simulink model "c00014M_harness"  (R2018a)
settings: Solver=FixedStepAuto  StartTime=0.0  StopTime=300  FixedStep=0.1  RelTol=1e-3
undefined symbols (not defined in the file): A1, hmax, PriorityTank, R1, R2, sigbuilder_block
(part 5 of 24)

== system c00014M_harness/M184 ==
  note: VALUES
      | ---------------------------------
      | ControlType = 1 | 2 | 3
      | FillTank = 0 | 1
      | EmptyTank = 0 | 1
      | ManualReference between 0 and 1
      | Tempreature between 0 and 100
      | EmergencyButton = 0 | 1
      | LiquidLevel between 0 and 1 (hmax)
  note: Inputs For Tank2
  note: NAMES
      | --------------------------------------------
      | CT1 = ControlType Tank 1
      | F1 = Fill Tank 1
      | E1 = Empty Tank 1
      | MR1 = Manual Reference Tank1
      | T1 = Temperature Tank 1
      | EB1 = Emergency Button Tank 1
      | LL1 = Liquid Level 1
  note: Inputs For Tank3
  note: Inputs For Tank1
  CT1 : Inport
  F1 : Inport  Port=2
  E1 : Inport  Port=3
  T1 : Inport  Port=4
  EB1 : Inport  Port=5
  CT3 : Inport  Port=6
  T3 : Inport  Port=7
  EB3 : Inport  Port=8
  Tank1 : Subsystem
  Tank3 : Subsystem
  LL1 : Outport
  LL3 : Outport  Port=2
  wires:
  EB1/1 -> Tank1/5(EB1)
  Tank3/1(LL3) -> LL3/1, Tank1/6(LL3)
  T1/1 -> Tank1/4(T1)
  Tank1/1(LL1) -> LL1/1, Tank3/4(LL1)
  F1/1 -> Tank1/2(F1)
  E1/1 -> Tank1/3(E1)
  CT3/1 -> Tank3/1(CT3)
  EB3/1 -> Tank3/3(EB3)
  T3/1 -> Tank3/2(T3)
  CT1/1 -> Tank1/1(CT1)

== system c00014M_harness/M185 ==
  note: VALUES
      | ---------------------------------
      | ControlType = 1 | 2 | 3
      | FillTank = 0 | 1
      | EmptyTank = 0 | 1
      | ManualReference between 0 and 1
      | Tempreature between 0 and 100
      | EmergencyButton = 0 | 1
      | LiquidLevel between 0 and 1 (hmax)
  note: Inputs For Tank2
  note: NAMES
      | --------------------------------------------
      | CT1 = ControlType Tank 1
      | F1 = Fill Tank 1
      | E1 = Empty Tank 1
      | MR1 = Manual Reference Tank1
      | T1 = Temperature Tank 1
      | EB1 = Emergency Button Tank 1
      | LL1 = Liquid Level 1
  note: Inputs For Tank3
  note: Inputs For Tank1
  CT1 : Inport
  F1 : Inport  Port=2
  E1 : Inport  Port=3
  T1 : Inport  Port=4
  EB1 : Inport  Port=5
  CT3 : Inport  Port=6
  T3 : Inport  Port=7
  EB3 : Inport  Port=8
  Tank1 : Subsystem
  Tank3 : Subsystem
  LL1 : Outport
  LL3 : Outport  Port=2
  wires:
  EB1/1 -> Tank1/5(EB1)
  Tank3/1(LL3) -> LL3/1, Tank1/6(LL3)
  T1/1 -> Tank1/4(T1)
  Tank1/1(LL1) -> LL1/1, Tank3/4(LL1)
  F1/1 -> Tank1/2(F1)
  E1/1 -> Tank1/3(E1)
  CT3/1 -> Tank3/1(CT3)
  EB3/1 -> Tank3/3(EB3)
  T3/1 -> Tank3/2(T3)
  CT1/1 -> Tank1/1(CT1)

== system c00014M_harness/M186 ==
  note: VALUES
      | ---------------------------------
      | ControlType = 1 | 2 | 3
      | FillTank = 0 | 1
      | EmptyTank = 0 | 1
      | ManualReference between 0 and 1
      | Tempreature between 0 and 100
      | EmergencyButton = 0 | 1
      | LiquidLevel between 0 and 1 (hmax)
  note: Inputs For Tank2
  note: NAMES
      | --------------------------------------------
      | CT1 = ControlType Tank 1
      | F1 = Fill Tank 1
      | E1 = Empty Tank 1
      | MR1 = Manual Reference Tank1
      | T1 = Temperature Tank 1
      | EB1 = Emergency Button Tank 1
      | LL1 = Liquid Level 1
  note: Inputs For Tank3
  note: Inputs For Tank1
  CT1 : Inport
  F1 : Inport  Port=2
  E1 : Inport  Port=3
  T1 : Inport  Port=4
  EB1 : Inport  Port=5
  CT3 : Inport  Port=6
  T3 : Inport  Port=7
  EB3 : Inport  Port=8
  Tank1 : Subsystem
  Tank3 : Subsystem
  LL1 : Outport
  LL3 : Outport  Port=2
  wires:
  EB1/1 -> Tank1/5(EB1)
  Tank3/1(LL3) -> LL3/1, Tank1/6(LL3)
  T1/1 -> Tank1/4(T1)
  Tank1/1(LL1) -> LL1/1, Tank3/4(LL1)
  F1/1 -> Tank1/2(F1)
  E1/1 -> Tank1/3(E1)
  CT3/1 -> Tank3/1(CT3)
  EB3/1 -> Tank3/3(EB3)
  T3/1 -> Tank3/2(T3)
  CT1/1 -> Tank1/1(CT1)

== system c00014M_harness/M187 ==
  note: VALUES
      | ---------------------------------
      | ControlType = 1 | 2 | 3
      | FillTank = 0 | 1
      | EmptyTank = 0 | 1
      | ManualReference between 0 and 1
      | Tempreature between 0 and 100
      | EmergencyButton = 0 | 1
      | LiquidLevel between 0 and 1 (hmax)
  note: Inputs For Tank2
  note: NAMES
      | --------------------------------------------
      | CT1 = ControlType Tank 1
      | F1 = Fill Tank 1
      | E1 = Empty Tank 1
      | MR1 = Manual Reference Tank1
      | T1 = Temperature Tank 1
      | EB1 = Emergency Button Tank 1
      | LL1 = Liquid Level 1
  note: Inputs For Tank3
  note: Inputs For Tank1
  CT1 : Inport
  F1 : Inport  Port=2
  E1 : Inport  Port=3
  T1 : Inport  Port=4
  EB1 : Inport  Port=5
  CT3 : Inport  Port=6
  T3 : Inport  Port=7
  EB3 : Inport  Port=8
  Tank1 : Subsystem
  Tank3 : Subsystem
  LL1 : Outport
  LL3 : Outport  Port=2
  wires:
  EB1/1 -> Tank1/5(EB1)
  Tank3/1(LL3) -> LL3/1, Tank1/6(LL3)
  T1/1 -> Tank1/4(T1)
  Tank1/1(LL1) -> LL1/1, Tank3/4(LL1)
  F1/1 -> Tank1/2(F1)
  E1/1 -> Tank1/3(E1)
  CT3/1 -> Tank3/1(CT3)
  EB3/1 -> Tank3/3(EB3)
  T3/1 -> Tank3/2(T3)
  CT1/1 -> Tank1/1(CT1)

== system c00014M_harness/M188 ==
  note: VALUES
      | ---------------------------------
      | ControlType = 1 | 2 | 3
      | FillTank = 0 | 1
      | EmptyTank = 0 | 1
      | ManualReference between 0 and 1
      | Tempreature between 0 and 100
      | EmergencyButton = 0 | 1
      | LiquidLevel between 0 and 1 (hmax)
  note: Inputs For Tank2
  note: NAMES
      | --------------------------------------------
      | CT1 = ControlType Tank 1
      | F1 = Fill Tank 1
      | E1 = Empty Tank 1
      | MR1 = Manual Reference Tank1
      | T1 = Temperature Tank 1
      | EB1 = Emergency Button Tank 1
      | LL1 = Liquid Level 1
  note: Inputs For Tank3
  note: Inputs For Tank1
  CT1 : Inport
  F1 : Inport  Port=2
  E1 : Inport  Port=3
  T1 : Inport  Port=4
  EB1 : Inport  Port=5
  CT3 : Inport  Port=6
  T3 : Inport  Port=7
  EB3 : Inport  Port=8
  Tank1 : Subsystem
  Tank3 : Subsystem
  LL1 : Outport
  LL3 : Outport  Port=2
  wires:
  EB1/1 -> Tank1/5(EB1)
  Tank3/1(LL3) -> LL3/1, Tank1/6(LL3)
  T1/1 -> Tank1/4(T1)
  Tank1/1(LL1) -> LL1/1, Tank3/4(LL1)
  F1/1 -> Tank1/2(F1)
  E1/1 -> Tank1/3(E1)
  CT3/1 -> Tank3/1(CT3)
  EB3/1 -> Tank3/3(EB3)
  T3/1 -> Tank3/2(T3)
  CT1/1 -> Tank1/1(CT1)

== system c00014M_harness/M189 ==
  note: VALUES
      | ---------------------------------
      | ControlType = 1 | 2 | 3
      | FillTank = 0 | 1
      | EmptyTank = 0 | 1
      | ManualReference between 0 and 1
      | Tempreature between 0 and 100
      | EmergencyButton = 0 | 1
      | LiquidLevel between 0 and 1 (hmax)
  note: Inputs For Tank2
  note: NAMES
      | --------------------------------------------
      | CT1 = ControlType Tank 1
      | F1 = Fill Tank 1
      | E1 = Empty Tank 1
      | MR1 = Manual Reference Tank1
      | T1 = Temperature Tank 1
      | EB1 = Emergency Button Tank 1
      | LL1 = Liquid Level 1
  note: Inputs For Tank3
  note: Inputs For Tank1
  CT1 : Inport
  F1 : Inport  Port=2
  E1 : Inport  Port=3
  T1 : Inport  Port=4
  EB1 : Inport  Port=5
  CT3 : Inport  Port=6
  T3 : Inport  Port=7
  EB3 : Inport  Port=8
  Tank1 : Subsystem
  Tank3 : Subsystem
  LL1 : Outport
  LL3 : Outport  Port=2
  wires:
  EB1/1 -> Tank1/5(EB1)
  Tank3/1(LL3) -> LL3/1, Tank1/6(LL3)
  T1/1 -> Tank1/4(T1)
  Tank1/1(LL1) -> LL1/1, Tank3/4(LL1)
  F1/1 -> Tank1/2(F1)
  E1/1 -> Tank1/3(E1)
  CT3/1 -> Tank3/1(CT3)
  EB3/1 -> Tank3/3(EB3)
  T3/1 -> Tank3/2(T3)
  CT1/1 -> Tank1/1(CT1)

== system c00014M_harness/M190 ==
  note: VALUES
      | ---------------------------------
      | ControlType = 1 | 2 | 3
      | FillTank = 0 | 1
      | EmptyTank = 0 | 1
      | ManualReference between 0 and 1
      | Tempreature between 0 and 100
      | EmergencyButton = 0 | 1
      | LiquidLevel between 0 and 1 (hmax)
  note: Inputs For Tank2
  note: NAMES
      | --------------------------------------------
      | CT1 = ControlType Tank 1
      | F1 = Fill Tank 1
      | E1 = Empty Tank 1
      | MR1 = Manual Reference Tank1
      | T1 = Temperature Tank 1
      | EB1 = Emergency Button Tank 1
      | LL1 = Liquid Level 1
  note: Inputs For Tank3
  note: Inputs For Tank1
  CT1 : Inport
  F1 : Inport  Port=2
  E1 : Inport  Port=3
  T1 : Inport  Port=4
  EB1 : Inport  Port=5
  CT3 : Inport  Port=6
  T3 : Inport  Port=7
  EB3 : Inport  Port=8
  Tank1 : Subsystem
  Tank3 : Subsystem
  LL1 : Outport
  LL3 : Outport  Port=2
  wires:
  EB1/1 -> Tank1/5(EB1)
  Tank3/1(LL3) -> LL3/1, Tank1/6(LL3)
  T1/1 -> Tank1/4(T1)
  Tank1/1(LL1) -> LL1/1, Tank3/4(LL1)
  F1/1 -> Tank1/2(F1)
  E1/1 -> Tank1/3(E1)
  CT3/1 -> Tank3/1(CT3)
  EB3/1 -> Tank3/3(EB3)
  T3/1 -> Tank3/2(T3)
  CT1/1 -> Tank1/1(CT1)

== system c00014M_harness/M191 ==
  note: VALUES
      | ---------------------------------
      | ControlType = 1 | 2 | 3
      | FillTank = 0 | 1
      | EmptyTank = 0 | 1
      | ManualReference between 0 and 1
      | Tempreature between 0 and 100
      | EmergencyButton = 0 | 1
      | LiquidLevel between 0 and 1 (hmax)
  note: Inputs For Tank2
  note: NAMES
      | --------------------------------------------
      | CT1 = ControlType Tank 1
      | F1 = Fill Tank 1
      | E1 = Empty Tank 1
      | MR1 = Manual Reference Tank1
      | T1 = Temperature Tank 1
      | EB1 = Emergency Button Tank 1
      | LL1 = Liquid Level 1
  note: Inputs For Tank3
  note: Inputs For Tank1
  CT1 : Inport
  F1 : Inport  Port=2
  E1 : Inport  Port=3
  T1 : Inport  Port=4
  EB1 : Inport  Port=5
  CT3 : Inport  Port=6
  T3 : Inport  Port=7
  EB3 : Inport  Port=8
  Tank1 : Subsystem
  Tank3 : Subsystem
  LL1 : Outport
  LL3 : Outport  Port=2
  wires:
  EB1/1 -> Tank1/5(EB1)
  Tank3/1(LL3) -> LL3/1, Tank1/6(LL3)
  T1/1 -> Tank1/4(T1)
  Tank1/1(LL1) -> LL1/1, Tank3/4(LL1)
  F1/1 -> Tank1/2(F1)
  E1/1 -> Tank1/3(E1)
  CT3/1 -> Tank3/1(CT3)
  EB3/1 -> Tank3/3(EB3)
  T3/1 -> Tank3/2(T3)
  CT1/1 -> Tank1/1(CT1)

== system c00014M_harness/M192 ==
  note: VALUES
      | ---------------------------------
      | ControlType = 1 | 2 | 3
      | FillTank = 0 | 1
      | EmptyTank = 0 | 1
      | ManualReference between 0 and 1
      | Tempreature between 0 and 100
      | EmergencyButton = 0 | 1
      | LiquidLevel between 0 and 1 (hmax)
  note: Inputs For Tank2
  note: NAMES
      | --------------------------------------------
      | CT1 = ControlType Tank 1
      | F1 = Fill Tank 1
      | E1 = Empty Tank 1
      | MR1 = Manual Reference Tank1
      | T1 = Temperature Tank 1
      | EB1 = Emergency Button Tank 1
      | LL1 = Liquid Level 1
  note: Inputs For Tank3
  note: Inputs For Tank1
  CT1 : Inport
  F1 : Inport  Port=2
  E1 : Inport  Port=3
  T1 : Inport  Port=4
  EB1 : Inport  Port=5
  CT3 : Inport  Port=6
  T3 : Inport  Port=7
  EB3 : Inport  Port=8
  Tank1 : Subsystem
  Tank3 : Subsystem
  LL1 : Outport
  LL3 : Outport  Port=2
  wires:
  EB1/1 -> Tank1/5(EB1)
  Tank3/1(LL3) -> LL3/1, Tank1/6(LL3)
  T1/1 -> Tank1/4(T1)
  Tank1/1(LL1) -> LL1/1, Tank3/4(LL1)
  F1/1 -> Tank1/2(F1)
  E1/1 -> Tank1/3(E1)
  CT3/1 -> Tank3/1(CT3)
  EB3/1 -> Tank3/3(EB3)
  T3/1 -> Tank3/2(T3)
  CT1/1 -> Tank1/1(CT1)

== system c00014M_harness/M193 ==
  note: VALUES
      | ---------------------------------
      | ControlType = 1 | 2 | 3
      | FillTank = 0 | 1
      | EmptyTank = 0 | 1
      | ManualReference between 0 and 1
      | Tempreature between 0 and 100
      | EmergencyButton = 0 | 1
      | LiquidLevel between 0 and 1 (hmax)
  note: Inputs For Tank2
  note: NAMES
      | --------------------------------------------
      | CT1 = ControlType Tank 1
      | F1 = Fill Tank 1
      | E1 = Empty Tank 1
      | MR1 = Manual Reference Tank1
      | T1 = Temperature Tank 1
      | EB1 = Emergency Button Tank 1
      | LL1 = Liquid Level 1
  note: Inputs For Tank3
  note: Inputs For Tank1
  CT1 : Inport
  F1 : Inport  Port=2
  E1 : Inport  Port=3
  T1 : Inport  Port=4
  EB1 : Inport  Port=5
  CT3 : Inport  Port=6
  T3 : Inport  Port=7
  EB3 : Inport  Port=8
  Tank1 : Subsystem
  Tank3 : Subsystem
  LL1 : Outport
  LL3 : Outport  Port=2
  wires:
  EB1/1 -> Tank1/5(EB1)
  Tank3/1(LL3) -> LL3/1, Tank1/6(LL3)
  T1/1 -> Tank1/4(T1)
  Tank1/1(LL1) -> LL1/1, Tank3/4(LL1)
  F1/1 -> Tank1/2(F1)
  E1/1 -> Tank1/3(E1)
  CT3/1 -> Tank3/1(CT3)
  EB3/1 -> Tank3/3(EB3)
  T3/1 -> Tank3/2(T3)
  CT1/1 -> Tank1/1(CT1)

== system c00014M_harness/M194 ==
  note: VALUES
      | ---------------------------------
      | ControlType = 1 | 2 | 3
      | FillTank = 0 | 1
      | EmptyTank = 0 | 1
      | ManualReference between 0 and 1
      | Tempreature between 0 and 100
      | EmergencyButton = 0 | 1
      | LiquidLevel between 0 and 1 (hmax)
  note: Inputs For Tank2
  note: NAMES
      | --------------------------------------------
      | CT1 = ControlType Tank 1
      | F1 = Fill Tank 1
      | E1 = Empty Tank 1
      | MR1 = Manual Reference Tank1
      | T1 = Temperature Tank 1
      | EB1 = Emergency Button Tank 1
      | LL1 = Liquid Level 1
  note: Inputs For Tank3
  note: Inputs For Tank1
  CT1 : Inport
  F1 : Inport  Port=2
  E1 : Inport  Port=3
  T1 : Inport  Port=4
  EB1 : Inport  Port=5
  CT3 : Inport  Port=6
  T3 : Inport  Port=7
  EB3 : Inport  Port=8
  Tank1 : Subsystem
  Tank3 : Subsystem
  LL1 : Outport
  LL3 : Outport  Port=2
  wires:
  EB1/1 -> Tank1/5(EB1)
  Tank3/1(LL3) -> LL3/1, Tank1/6(LL3)
  T1/1 -> Tank1/4(T1)
  Tank1/1(LL1) -> LL1/1, Tank3/4(LL1)
  F1/1 -> Tank1/2(F1)
  E1/1 -> Tank1/3(E1)
  CT3/1 -> Tank3/1(CT3)
  EB3/1 -> Tank3/3(EB3)
  T3/1 -> Tank3/2(T3)
  CT1/1 -> Tank1/1(CT1)

== system c00014M_harness/M195 ==
  note: VALUES
      | ---------------------------------
      | ControlType = 1 | 2 | 3
      | FillTank = 0 | 1
      | EmptyTank = 0 | 1
      | ManualReference between 0 and 1
      | Tempreature between 0 and 100
      | EmergencyButton = 0 | 1
      | LiquidLevel between 0 and 1 (hmax)
  note: Inputs For Tank2
  note: NAMES
      | --------------------------------------------
      | CT1 = ControlType Tank 1
      | F1 = Fill Tank 1
      | E1 = Empty Tank 1
      | MR1 = Manual Reference Tank1
      | T1 = Temperature Tank 1
      | EB1 = Emergency Button Tank 1
      | LL1 = Liquid Level 1
  note: Inputs For Tank3
  note: Inputs For Tank1
  CT1 : Inport
  F1 : Inport  Port=2
  E1 : Inport  Port=3
  T1 : Inport  Port=4
  EB1 : Inport  Port=5
  CT3 : Inport  Port=6
  T3 : Inport  Port=7
  EB3 : Inport  Port=8
  Tank1 : Subsystem
  Tank3 : Subsystem
  LL1 : Outport
  LL3 : Outport  Port=2
  wires:
  EB1/1 -> Tank1/5(EB1)
  Tank3/1(LL3) -> LL3/1, Tank1/6(LL3)
  T1/1 -> Tank1/4(T1)
  Tank1/1(LL1) -> LL1/1, Tank3/4(LL1)
  F1/1 -> Tank1/2(F1)
  E1/1 -> Tank1/3(E1)
  CT3/1 -> Tank3/1(CT3)
  EB3/1 -> Tank3/3(EB3)
  T3/1 -> Tank3/2(T3)
  CT1/1 -> Tank1/1(CT1)

== system c00014M_harness/M196 ==
  note: VALUES
      | ---------------------------------
      | ControlType = 1 | 2 | 3
      | FillTank = 0 | 1
      | EmptyTank = 0 | 1
      | ManualReference between 0 and 1
      | Tempreature between 0 and 100
      | EmergencyButton = 0 | 1
      | LiquidLevel between 0 and 1 (hmax)
  note: Inputs For Tank2
  note: NAMES
      | --------------------------------------------
      | CT1 = ControlType Tank 1
      | F1 = Fill Tank 1
      | E1 = Empty Tank 1
      | MR1 = Manual Reference Tank1
      | T1 = Temperature Tank 1
      | EB1 = Emergency Button Tank 1
      | LL1 = Liquid Level 1
  note: Inputs For Tank3
  note: Inputs For Tank1
  CT1 : Inport
  F1 : Inport  Port=2
  E1 : Inport  Port=3
  T1 : Inport  Port=4
  EB1 : Inport  Port=5
  CT3 : Inport  Port=6
  T3 : Inport  Port=7
  EB3 : Inport  Port=8
  Tank1 : Subsystem
  Tank3 : Subsystem
  LL1 : Outport
  LL3 : Outport  Port=2
  wires:
  EB1/1 -> Tank1/5(EB1)
  Tank3/1(LL3) -> LL3/1, Tank1/6(LL3)
  T1/1 -> Tank1/4(T1)
  Tank1/1(LL1) -> LL1/1, Tank3/4(LL1)
  F1/1 -> Tank1/2(F1)
  E1/1 -> Tank1/3(E1)
  CT3/1 -> Tank3/1(CT3)
  EB3/1 -> Tank3/3(EB3)
  T3/1 -> Tank3/2(T3)
  CT1/1 -> Tank1/1(CT1)

== system c00014M_harness/M197 ==
  note: VALUES
      | ---------------------------------
      | ControlType = 1 | 2 | 3
      | FillTank = 0 | 1
      | EmptyTank = 0 | 1
      | ManualReference between 0 and 1
      | Tempreature between 0 and 100
      | EmergencyButton = 0 | 1
      | LiquidLevel between 0 and 1 (hmax)
  note: Inputs For Tank2
  note: NAMES
      | --------------------------------------------
      | CT1 = ControlType Tank 1
      | F1 = Fill Tank 1
      | E1 = Empty Tank 1
      | MR1 = Manual Reference Tank1
      | T1 = Temperature Tank 1
      | EB1 = Emergency Button Tank 1
      | LL1 = Liquid Level 1
  note: Inputs For Tank3
  note: Inputs For Tank1
  CT1 : Inport
  F1 : Inport  Port=2
  E1 : Inport  Port=3
  T1 : Inport  Port=4
  EB1 : Inport  Port=5
  CT3 : Inport  Port=6
  T3 : Inport  Port=7
  EB3 : Inport  Port=8
  Tank1 : Subsystem
  Tank3 : Subsystem
  LL1 : Outport
  LL3 : Outport  Port=2
  wires:
  EB1/1 -> Tank1/5(EB1)
  Tank3/1(LL3) -> LL3/1, Tank1/6(LL3)
  T1/1 -> Tank1/4(T1)
  Tank1/1(LL1) -> LL1/1, Tank3/4(LL1)
  F1/1 -> Tank1/2(F1)
  E1/1 -> Tank1/3(E1)
  CT3/1 -> Tank3/1(CT3)
  EB3/1 -> Tank3/3(EB3)
  T3/1 -> Tank3/2(T3)
  CT1/1 -> Tank1/1(CT1)

== system c00014M_harness/M198 ==
  note: VALUES
      | ---------------------------------
      | ControlType = 1 | 2 | 3
      | FillTank = 0 | 1
      | EmptyTank = 0 | 1
      | ManualReference between 0 and 1
      | Tempreature between 0 and 100
      | EmergencyButton = 0 | 1
      | LiquidLevel between 0 and 1 (hmax)
  note: Inputs For Tank2
  note: NAMES
      | --------------------------------------------
      | CT1 = ControlType Tank 1
      | F1 = Fill Tank 1
      | E1 = Empty Tank 1
      | MR1 = Manual Reference Tank1
      | T1 = Temperature Tank 1
      | EB1 = Emergency Button Tank 1
      | LL1 = Liquid Level 1
  note: Inputs For Tank3
  note: Inputs For Tank1
  CT1 : Inport
  F1 : Inport  Port=2
  E1 : Inport  Port=3
  T1 : Inport  Port=4
  EB1 : Inport  Port=5
  CT3 : Inport  Port=6
  T3 : Inport  Port=7
  EB3 : Inport  Port=8
  Tank1 : Subsystem
  Tank3 : Subsystem
  LL1 : Outport
  LL3 : Outport  Port=2
  wires:
  EB1/1 -> Tank1/5(EB1)
  Tank3/1(LL3) -> LL3/1, Tank1/6(LL3)
  T1/1 -> Tank1/4(T1)
  Tank1/1(LL1) -> LL1/1, Tank3/4(LL1)
  F1/1 -> Tank1/2(F1)
  E1/1 -> Tank1/3(E1)
  CT3/1 -> Tank3/1(CT3)
  EB3/1 -> Tank3/3(EB3)
  T3/1 -> Tank3/2(T3)
  CT1/1 -> Tank1/1(CT1)

== system c00014M_harness/M199 ==
  note: VALUES
      | ---------------------------------
      | ControlType = 1 | 2 | 3
      | FillTank = 0 | 1
      | EmptyTank = 0 | 1
      | ManualReference between 0 and 1
      | Tempreature between 0 and 100
      | EmergencyButton = 0 | 1
      | LiquidLevel between 0 and 1 (hmax)
  note: Inputs For Tank2
  note: NAMES
      | --------------------------------------------
      | CT1 = ControlType Tank 1
      | F1 = Fill Tank 1
      | E1 = Empty Tank 1
      | MR1 = Manual Reference Tank1
      | T1 = Temperature Tank 1
      | EB1 = Emergency Button Tank 1
      | LL1 = Liquid Level 1
  note: Inputs For Tank3
  note: Inputs For Tank1
  CT1 : Inport
  F1 : Inport  Port=2
  E1 : Inport  Port=3
  T1 : Inport  Port=4
  EB1 : Inport  Port=5
  CT3 : Inport  Port=6
  T3 : Inport  Port=7
  EB3 : Inport  Port=8
  Tank1 : Subsystem
  Tank3 : Subsystem
  LL1 : Outport
  LL3 : Outport  Port=2
  wires:
  EB1/1 -> Tank1/5(EB1)
  Tank3/1(LL3) -> LL3/1, Tank1/6(LL3)
  T1/1 -> Tank1/4(T1)
  Tank1/1(LL1) -> LL1/1, Tank3/4(LL1)
  F1/1 -> Tank1/2(F1)
  E1/1 -> Tank1/3(E1)
  CT3/1 -> Tank3/1(CT3)
  EB3/1 -> Tank3/3(EB3)
  T3/1 -> Tank3/2(T3)
  CT1/1 -> Tank1/1(CT1)

== system c00014M_harness/M222 ==
  note: VALUES
      | ---------------------------------
      | ControlType = 1 | 2 | 3
      | FillTank = 0 | 1
      | EmptyTank = 0 | 1
      | ManualReference between 0 and 1
      | Tempreature between 0 and 100
      | EmergencyButton = 0 | 1
      | LiquidLevel between 0 and 1 (hmax)
  note: Inputs For Tank2
  note: NAMES
      | --------------------------------------------
      | CT1 = ControlType Tank 1
      | F1 = Fill Tank 1
      | E1 = Empty Tank 1
      | MR1 = Manual Reference Tank1
      | T1 = Temperature Tank 1
      | EB1 = Emergency Button Tank 1
      | LL1 = Liquid Level 1
  note: Inputs For Tank3
  note: Inputs For Tank1
  CT1 : Inport
  F1 : Inport  Port=2
  E1 : Inport  Port=3
  T1 : Inport  Port=4
  EB1 : Inport  Port=5
  CT3 : Inport  Port=6
  T3 : Inport  Port=7
  EB3 : Inport  Port=8
  Tank1 : Subsystem
  Tank3 : Subsystem
  LL1 : Outport
  LL3 : Outport  Port=2
  wires:
  EB1/1 -> Tank1/5(EB1)
  Tank3/1(LL3) -> LL3/1, Tank1/6(LL3)
  T1/1 -> Tank1/4(T1)
  Tank1/1(LL1) -> LL1/1, Tank3/4(LL1)
  F1/1 -> Tank1/2(F1)
  E1/1 -> Tank1/3(E1)
  CT3/1 -> Tank3/1(CT3)
  EB3/1 -> Tank3/3(EB3)
  T3/1 -> Tank3/2(T3)
  CT1/1 -> Tank1/1(CT1)

== system c00014M_harness/M223 ==
  note: VALUES
      | ---------------------------------
      | ControlType = 1 | 2 | 3
      | FillTank = 0 | 1
      | EmptyTank = 0 | 1
      | ManualReference between 0 and 1
      | Tempreature between 0 and 100
      | EmergencyButton = 0 | 1
      | LiquidLevel between 0 and 1 (hmax)
  note: Inputs For Tank2
  note: NAMES
      | --------------------------------------------
      | CT1 = ControlType Tank 1
      | F1 = Fill Tank 1
      | E1 = Empty Tank 1
      | MR1 = Manual Reference Tank1
      | T1 = Temperature Tank 1
      | EB1 = Emergency Button Tank 1
      | LL1 = Liquid Level 1
  note: Inputs For Tank3
  note: Inputs For Tank1
  CT1 : Inport
  F1 : Inport  Port=2
  E1 : Inport  Port=3
  T1 : Inport  Port=4
  EB1 : Inport  Port=5
  CT3 : Inport  Port=6
  T3 : Inport  Port=7
  EB3 : Inport  Port=8
  Tank1 : Subsystem
  Tank3 : Subsystem
  LL1 : Outport
  LL3 : Outport  Port=2
  wires:
  EB1/1 -> Tank1/5(EB1)
  Tank3/1(LL3) -> LL3/1, Tank1/6(LL3)
  T1/1 -> Tank1/4(T1)
  Tank1/1(LL1) -> LL1/1, Tank3/4(LL1)
  F1/1 -> Tank1/2(F1)
  E1/1 -> Tank1/3(E1)
  CT3/1 -> Tank3/1(CT3)
  EB3/1 -> Tank3/3(EB3)
  T3/1 -> Tank3/2(T3)
  CT1/1 -> Tank1/1(CT1)

== system c00014M_harness/M224 ==
  note: VALUES
      | ---------------------------------
      | ControlType = 1 | 2 | 3
      | FillTank = 0 | 1
      | EmptyTank = 0 | 1
      | ManualReference between 0 and 1
      | Tempreature between 0 and 100
      | EmergencyButton = 0 | 1
      | LiquidLevel between 0 and 1 (hmax)
  note: Inputs For Tank2
  note: NAMES
      | --------------------------------------------
      | CT1 = ControlType Tank 1
      | F1 = Fill Tank 1
      | E1 = Empty Tank 1
      | MR1 = Manual Reference Tank1
      | T1 = Temperature Tank 1
      | EB1 = Emergency Button Tank 1
      | LL1 = Liquid Level 1
  note: Inputs For Tank3
  note: Inputs For Tank1
  CT1 : Inport
  F1 : Inport  Port=2
  E1 : Inport  Port=3
  T1 : Inport  Port=4
  EB1 : Inport  Port=5
  CT3 : Inport  Port=6
  T3 : Inport  Port=7
  EB3 : Inport  Port=8
  Tank1 : Subsystem
  Tank3 : Subsystem
  LL1 : Outport
  LL3 : Outport  Port=2
  wires:
  EB1/1 -> Tank1/5(EB1)
  Tank3/1(LL3) -> LL3/1, Tank1/6(LL3)
  T1/1 -> Tank1/4(T1)
  Tank1/1(LL1) -> LL1/1, Tank3/4(LL1)
  F1/1 -> Tank1/2(F1)
  E1/1 -> Tank1/3(E1)
  CT3/1 -> Tank3/1(CT3)
  EB3/1 -> Tank3/3(EB3)
  T3/1 -> Tank3/2(T3)
  CT1/1 -> Tank1/1(CT1)

== system c00014M_harness/M225 ==
  note: VALUES
      | ---------------------------------
      | ControlType = 1 | 2 | 3
      | FillTank = 0 | 1
      | EmptyTank = 0 | 1
      | ManualReference between 0 and 1
      | Tempreature between 0 and 100
      | EmergencyButton = 0 | 1
      | LiquidLevel between 0 and 1 (hmax)
  note: Inputs For Tank2
  note: NAMES
      | --------------------------------------------
      | CT1 = ControlType Tank 1
      | F1 = Fill Tank 1
      | E1 = Empty Tank 1
      | MR1 = Manual Reference Tank1
      | T1 = Temperature Tank 1
      | EB1 = Emergency Button Tank 1
      | LL1 = Liquid Level 1
  note: Inputs For Tank3
  note: Inputs For Tank1
  CT1 : Inport
  F1 : Inport  Port=2
  E1 : Inport  Port=3
  T1 : Inport  Port=4
  EB1 : Inport  Port=5
  CT3 : Inport  Port=6
  T3 : Inport  Port=7
  EB3 : Inport  Port=8
  Tank1 : Subsystem
  Tank3 : Subsystem
  LL1 : Outport
  LL3 : Outport  Port=2
  wires:
  EB1/1 -> Tank1/5(EB1)
  Tank3/1(LL3) -> LL3/1, Tank1/6(LL3)
  T1/1 -> Tank1/4(T1)
  Tank1/1(LL1) -> LL1/1, Tank3/4(LL1)
  F1/1 -> Tank1/2(F1)
  E1/1 -> Tank1/3(E1)
  CT3/1 -> Tank3/1(CT3)
  EB3/1 -> Tank3/3(EB3)
  T3/1 -> Tank3/2(T3)
  CT1/1 -> Tank1/1(CT1)

== system c00014M_harness/M226 ==
  note: VALUES
      | ---------------------------------
      | ControlType = 1 | 2 | 3
      | FillTank = 0 | 1
      | EmptyTank = 0 | 1
      | ManualReference between 0 and 1
      | Tempreature between 0 and 100
      | EmergencyButton = 0 | 1
      | LiquidLevel between 0 and 1 (hmax)
  note: Inputs For Tank2
  note: NAMES
      | --------------------------------------------
      | CT1 = ControlType Tank 1
      | F1 = Fill Tank 1
      | E1 = Empty Tank 1
      | MR1 = Manual Reference Tank1
      | T1 = Temperature Tank 1
      | EB1 = Emergency Button Tank 1
      | LL1 = Liquid Level 1
  note: Inputs For Tank3
  note: Inputs For Tank1
  CT1 : Inport
  F1 : Inport  Port=2
  E1 : Inport  Port=3
  T1 : Inport  Port=4
  EB1 : Inport  Port=5
  CT3 : Inport  Port=6
  T3 : Inport  Port=7
  EB3 : Inport  Port=8
  Tank1 : Subsystem
  Tank3 : Subsystem
  LL1 : Outport
  LL3 : Outport  Port=2
  wires:
  EB1/1 -> Tank1/5(EB1)
  Tank3/1(LL3) -> LL3/1, Tank1/6(LL3)
  T1/1 -> Tank1/4(T1)
  Tank1/1(LL1) -> LL1/1, Tank3/4(LL1)
  F1/1 -> Tank1/2(F1)
  E1/1 -> Tank1/3(E1)
  CT3/1 -> Tank3/1(CT3)
  EB3/1 -> Tank3/3(EB3)
  T3/1 -> Tank3/2(T3)
  CT1/1 -> Tank1/1(CT1)

== system c00014M_harness/M227 ==
  note: VALUES
      | ---------------------------------
      | ControlType = 1 | 2 | 3
      | FillTank = 0 | 1
      | EmptyTank = 0 | 1
      | ManualReference between 0 and 1
      | Tempreature between 0 and 100
      | EmergencyButton = 0 | 1
      | LiquidLevel between 0 and 1 (hmax)
  note: Inputs For Tank2
  note: NAMES
      | --------------------------------------------
      | CT1 = ControlType Tank 1
      | F1 = Fill Tank 1
      | E1 = Empty Tank 1
      | MR1 = Manual Reference Tank1
      | T1 = Temperature Tank 1
      | EB1 = Emergency Button Tank 1
      | LL1 = Liquid Level 1
  note: Inputs For Tank3
  note: Inputs For Tank1
  CT1 : Inport
  F1 : Inport  Port=2
  E1 : Inport  Port=3
  T1 : Inport  Port=4
  EB1 : Inport  Port=5
  CT3 : Inport  Port=6
  T3 : Inport  Port=7
  EB3 : Inport  Port=8
  Tank1 : Subsystem
  Tank3 : Subsystem
  LL1 : Outport
  LL3 : Outport  Port=2
  wires:
  EB1/1 -> Tank1/5(EB1)
  Tank3/1(LL3) -> LL3/1, Tank1/6(LL3)
  T1/1 -> Tank1/4(T1)
  Tank1/1(LL1) -> LL1/1, Tank3/4(LL1)
  F1/1 -> Tank1/2(F1)
  E1/1 -> Tank1/3(E1)
  CT3/1 -> Tank3/1(CT3)
  EB3/1 -> Tank3/3(EB3)
  T3/1 -> Tank3/2(T3)
  CT1/1 -> Tank1/1(CT1)

== system c00014M_harness/M228 ==
  note: VALUES
      | ---------------------------------
      | ControlType = 1 | 2 | 3
      | FillTank = 0 | 1
      | EmptyTank = 0 | 1
      | ManualReference between 0 and 1
      | Tempreature between 0 and 100
      | EmergencyButton = 0 | 1
      | LiquidLevel between 0 and 1 (hmax)
  note: Inputs For Tank2
  note: NAMES
      | --------------------------------------------
      | CT1 = ControlType Tank 1
      | F1 = Fill Tank 1
      | E1 = Empty Tank 1
      | MR1 = Manual Reference Tank1
      | T1 = Temperature Tank 1
      | EB1 = Emergency Button Tank 1
      | LL1 = Liquid Level 1
  note: Inputs For Tank3
  note: Inputs For Tank1
  CT1 : Inport
  F1 : Inport  Port=2
  E1 : Inport  Port=3
  T1 : Inport  Port=4
  EB1 : Inport  Port=5
  CT3 : Inport  Port=6
  T3 : Inport  Port=7
  EB3 : Inport  Port=8
  Tank1 : Subsystem
  Tank3 : Subsystem
  LL1 : Outport
  LL3 : Outport  Port=2
  wires:
  EB1/1 -> Tank1/5(EB1)
  Tank3/1(LL3) -> LL3/1, Tank1/6(LL3)
  T1/1 -> Tank1/4(T1)
  Tank1/1(LL1) -> LL1/1, Tank3/4(LL1)
  F1/1 -> Tank1/2(F1)
  E1/1 -> Tank1/3(E1)
  CT3/1 -> Tank3/1(CT3)
  EB3/1 -> Tank3/3(EB3)
  T3/1 -> Tank3/2(T3)
  CT1/1 -> Tank1/1(CT1)

== system c00014M_harness/M229 ==
  note: VALUES
      | ---------------------------------
      | ControlType = 1 | 2 | 3
      | FillTank = 0 | 1
      | EmptyTank = 0 | 1
      | ManualReference between 0 and 1
      | Tempreature between 0 and 100
      | EmergencyButton = 0 | 1
      | LiquidLevel between 0 and 1 (hmax)
  note: Inputs For Tank2
  note: NAMES
      | --------------------------------------------
      | CT1 = ControlType Tank 1
      | F1 = Fill Tank 1
      | E1 = Empty Tank 1
      | MR1 = Manual Reference Tank1
      | T1 = Temperature Tank 1
      | EB1 = Emergency Button Tank 1
      | LL1 = Liquid Level 1
  note: Inputs For Tank3
  note: Inputs For Tank1
  CT1 : Inport
  F1 : Inport  Port=2
  E1 : Inport  Port=3
  T1 : Inport  Port=4
  EB1 : Inport  Port=5
  CT3 : Inport  Port=6
  T3 : Inport  Port=7
  EB3 : Inport  Port=8
  Tank1 : Subsystem
  Tank3 : Subsystem
  LL1 : Outport
  LL3 : Outport  Port=2
  wires:
  EB1/1 -> Tank1/5(EB1)
  Tank3/1(LL3) -> LL3/1, Tank1/6(LL3)
  T1/1 -> Tank1/4(T1)
  Tank1/1(LL1) -> LL1/1, Tank3/4(LL1)
  F1/1 -> Tank1/2(F1)
  E1/1 -> Tank1/3(E1)
  CT3/1 -> Tank3/1(CT3)
  EB3/1 -> Tank3/3(EB3)
  T3/1 -> Tank3/2(T3)
  CT1/1 -> Tank1/1(CT1)

== system c00014M_harness/M230 ==
  note: VALUES
      | ---------------------------------
      | ControlType = 1 | 2 | 3
      | FillTank = 0 | 1
      | EmptyTank = 0 | 1
      | ManualReference between 0 and 1
      | Tempreature between 0 and 100
      | EmergencyButton = 0 | 1
      | LiquidLevel between 0 and 1 (hmax)
  note: Inputs For Tank2
  note: NAMES
      | --------------------------------------------
      | CT1 = ControlType Tank 1
      | F1 = Fill Tank 1
      | E1 = Empty Tank 1
      | MR1 = Manual Reference Tank1
      | T1 = Temperature Tank 1
      | EB1 = Emergency Button Tank 1
      | LL1 = Liquid Level 1
  note: Inputs For Tank3
  note: Inputs For Tank1
  CT1 : Inport
  F1 : Inport  Port=2
  E1 : Inport  Port=3
  T1 : Inport  Port=4
  EB1 : Inport  Port=5
  CT3 : Inport  Port=6
  T3 : Inport  Port=7
  EB3 : Inport  Port=8
  Tank1 : Subsystem
  Tank3 : Subsystem
  LL1 : Outport
  LL3 : Outport  Port=2
  wires:
  EB1/1 -> Tank1/5(EB1)
  Tank3/1(LL3) -> LL3/1, Tank1/6(LL3)
  T1/1 -> Tank1/4(T1)
  Tank1/1(LL1) -> LL1/1, Tank3/4(LL1)
  F1/1 -> Tank1/2(F1)
  E1/1 -> Tank1/3(E1)
  CT3/1 -> Tank3/1(CT3)
  EB3/1 -> Tank3/3(EB3)
  T3/1 -> Tank3/2(T3)
  CT1/1 -> Tank1/1(CT1)

== system c00014M_harness/M231 ==
  note: VALUES
      | ---------------------------------
      | ControlType = 1 | 2 | 3
      | FillTank = 0 | 1
      | EmptyTank = 0 | 1
      | ManualReference between 0 and 1
      | Tempreature between 0 and 100
      | EmergencyButton = 0 | 1
      | LiquidLevel between 0 and 1 (hmax)
  note: Inputs For Tank2
  note: NAMES
      | --------------------------------------------
      | CT1 = ControlType Tank 1
      | F1 = Fill Tank 1
      | E1 = Empty Tank 1
      | MR1 = Manual Reference Tank1
      | T1 = Temperature Tank 1
      | EB1 = Emergency Button Tank 1
      | LL1 = Liquid Level 1
  note: Inputs For Tank3
  note: Inputs For Tank1
  CT1 : Inport
  F1 : Inport  Port=2
  E1 : Inport  Port=3
  T1 : Inport  Port=4
  EB1 : Inport  Port=5
  CT3 : Inport  Port=6
  T3 : Inport  Port=7
  EB3 : Inport  Port=8
  Tank1 : Subsystem
  Tank3 : Subsystem
  LL1 : Outport
  LL3 : Outport  Port=2
  wires:
  EB1/1 -> Tank1/5(EB1)
  Tank3/1(LL3) -> LL3/1, Tank1/6(LL3)
  T1/1 -> Tank1/4(T1)
  Tank1/1(LL1) -> LL1/1, Tank3/4(LL1)
  F1/1 -> Tank1/2(F1)
  E1/1 -> Tank1/3(E1)
  CT3/1 -> Tank3/1(CT3)
  EB3/1 -> Tank3/3(EB3)
  T3/1 -> Tank3/2(T3)
  CT1/1 -> Tank1/1(CT1)

== system c00014M_harness/M232 ==
  note: VALUES
      | ---------------------------------
      | ControlType = 1 | 2 | 3
      | FillTank = 0 | 1
      | EmptyTank = 0 | 1
      | ManualReference between 0 and 1
      | Tempreature between 0 and 100
      | EmergencyButton = 0 | 1
      | LiquidLevel between 0 and 1 (hmax)
  note: Inputs For Tank2
  note: NAMES
      | --------------------------------------------
      | CT1 = ControlType Tank 1
      | F1 = Fill Tank 1
      | E1 = Empty Tank 1
      | MR1 = Manual Reference Tank1
      | T1 = Temperature Tank 1
      | EB1 = Emergency Button Tank 1
      | LL1 = Liquid Level 1
  note: Inputs For Tank3
  note: Inputs For Tank1
  CT1 : Inport
  F1 : Inport  Port=2
  E1 : Inport  Port=3
  T1 : Inport  Port=4
  EB1 : Inport  Port=5
  CT3 : Inport  Port=6
  T3 : Inport  Port=7
  EB3 : Inport  Port=8
  Tank1 : Subsystem
  Tank3 : Subsystem
  LL1 : Outport
  LL3 : Outport  Port=2
  wires:
  EB1/1 -> Tank1/5(EB1)
  Tank3/1(LL3) -> LL3/1, Tank1/6(LL3)
  T1/1 -> Tank1/4(T1)
  Tank1/1(LL1) -> LL1/1, Tank3/4(LL1)
  F1/1 -> Tank1/2(F1)
  E1/1 -> Tank1/3(E1)
  CT3/1 -> Tank3/1(CT3)
  EB3/1 -> Tank3/3(EB3)
  T3/1 -> Tank3/2(T3)
  CT1/1 -> Tank1/1(CT1)

== system c00014M_harness/M233 ==
  note: VALUES
      | ---------------------------------
      | ControlType = 1 | 2 | 3
      | FillTank = 0 | 1
      | EmptyTank = 0 | 1
      | ManualReference between 0 and 1
      | Tempreature between 0 and 100
      | EmergencyButton = 0 | 1
      | LiquidLevel between 0 and 1 (hmax)
  note: Inputs For Tank2
  note: NAMES
      | --------------------------------------------
      | CT1 = ControlType Tank 1
      | F1 = Fill Tank 1
      | E1 = Empty Tank 1
      | MR1 = Manual Reference Tank1
      | T1 = Temperature Tank 1
      | EB1 = Emergency Button Tank 1
      | LL1 = Liquid Level 1
  note: Inputs For Tank3
  note: Inputs For Tank1
  CT1 : Inport
  F1 : Inport  Port=2
  E1 : Inport  Port=3
  T1 : Inport  Port=4
  EB1 : Inport  Port=5
  CT3 : Inport  Port=6
  T3 : Inport  Port=7
  EB3 : Inport  Port=8
  Tank1 : Subsystem
  Tank3 : Subsystem
  LL1 : Outport
  LL3 : Outport  Port=2
  wires:
  EB1/1 -> Tank1/5(EB1)
  Tank3/1(LL3) -> LL3/1, Tank1/6(LL3)
  T1/1 -> Tank1/4(T1)
  Tank1/1(LL1) -> LL1/1, Tank3/4(LL1)
  F1/1 -> Tank1/2(F1)
  E1/1 -> Tank1/3(E1)
  CT3/1 -> Tank3/1(CT3)
  EB3/1 -> Tank3/3(EB3)
  T3/1 -> Tank3/2(T3)
  CT1/1 -> Tank1/1(CT1)

== system c00014M_harness/M234 ==
  note: VALUES
      | ---------------------------------
      | ControlType = 1 | 2 | 3
      | FillTank = 0 | 1
      | EmptyTank = 0 | 1
      | ManualReference between 0 and 1
      | Tempreature between 0 and 100
      | EmergencyButton = 0 | 1
      | LiquidLevel between 0 and 1 (hmax)
  note: Inputs For Tank2
  note: NAMES
      | --------------------------------------------
      | CT1 = ControlType Tank 1
      | F1 = Fill Tank 1
      | E1 = Empty Tank 1
      | MR1 = Manual Reference Tank1
      | T1 = Temperature Tank 1
      | EB1 = Emergency Button Tank 1
      | LL1 = Liquid Level 1
  note: Inputs For Tank3
  note: Inputs For Tank1
  CT1 : Inport
  F1 : Inport  Port=2
  E1 : Inport  Port=3
  T1 : Inport  Port=4
  EB1 : Inport  Port=5
  CT3 : Inport  Port=6
  T3 : Inport  Port=7
  EB3 : Inport  Port=8
  Tank1 : Subsystem
  Tank3 : Subsystem
  LL1 : Outport
  LL3 : Outport  Port=2
  wires:
  EB1/1 -> Tank1/5(EB1)
  Tank3/1(LL3) -> LL3/1, Tank1/6(LL3)
  T1/1 -> Tank1/4(T1)
  Tank1/1(LL1) -> LL1/1, Tank3/4(LL1)
  F1/1 -> Tank1/2(F1)
  E1/1 -> Tank1/3(E1)
  CT3/1 -> Tank3/1(CT3)
  EB3/1 -> Tank3/3(EB3)
  T3/1 -> Tank3/2(T3)
  CT1/1 -> Tank1/1(CT1)

== system c00014M_harness/M235 ==
  note: VALUES
      | ---------------------------------
      | ControlType = 1 | 2 | 3
      | FillTank = 0 | 1
      | EmptyTank = 0 | 1
      | ManualReference between 0 and 1
      | Tempreature between 0 and 100
      | EmergencyButton = 0 | 1
      | LiquidLevel between 0 and 1 (hmax)
  note: Inputs For Tank2
  note: NAMES
      | --------------------------------------------
      | CT1 = ControlType Tank 1
      | F1 = Fill Tank 1
      | E1 = Empty Tank 1
      | MR1 = Manual Reference Tank1
      | T1 = Temperature Tank 1
      | EB1 = Emergency Button Tank 1
      | LL1 = Liquid Level 1
  note: Inputs For Tank3
  note: Inputs For Tank1
  CT1 : Inport
  F1 : Inport  Port=2
  E1 : Inport  Port=3
  T1 : Inport  Port=4
  EB1 : Inport  Port=5
  CT3 : Inport  Port=6
  T3 : Inport  Port=7
  EB3 : Inport  Port=8
  Tank1 : Subsystem
  Tank3 : Subsystem
  LL1 : Outport
  LL3 : Outport  Port=2
  wires:
  EB1/1 -> Tank1/5(EB1)
  Tank3/1(LL3) -> LL3/1, Tank1/6(LL3)
  T1/1 -> Tank1/4(T1)
  Tank1/1(LL1) -> LL1/1, Tank3/4(LL1)
  F1/1 -> Tank1/2(F1)
  E1/1 -> Tank1/3(E1)
  CT3/1 -> Tank3/1(CT3)
  EB3/1 -> Tank3/3(EB3)
  T3/1 -> Tank3/2(T3)
  CT1/1 -> Tank1/1(CT1)

== system c00014M_harness/M236 ==
  note: VALUES
      | ---------------------------------
      | ControlType = 1 | 2 | 3
      | FillTank = 0 | 1
      | EmptyTank = 0 | 1
      | ManualReference between 0 and 1
      | Tempreature between 0 and 100
      | EmergencyButton = 0 | 1
      | LiquidLevel between 0 and 1 (hmax)
  note: Inputs For Tank2
  note: NAMES
      | --------------------------------------------
      | CT1 = ControlType Tank 1
      | F1 = Fill Tank 1
      | E1 = Empty Tank 1
      | MR1 = Manual Reference Tank1
      | T1 = Temperature Tank 1
      | EB1 = Emergency Button Tank 1
      | LL1 = Liquid Level 1
  note: Inputs For Tank3
  note: Inputs For Tank1
  CT1 : Inport
  F1 : Inport  Port=2
  E1 : Inport  Port=3
  T1 : Inport  Port=4
  EB1 : Inport  Port=5
  CT3 : Inport  Port=6
  T3 : Inport  Port=7
  EB3 : Inport  Port=8
  Tank1 : Subsystem
  Tank3 : Subsystem
  LL1 : Outport
  LL3 : Outport  Port=2
  wires:
  EB1/1 -> Tank1/5(EB1)
  Tank3/1(LL3) -> LL3/1, Tank1/6(LL3)
  T1/1 -> Tank1/4(T1)
  Tank1/1(LL1) -> LL1/1, Tank3/4(LL1)
  F1/1 -> Tank1/2(F1)
  E1/1 -> Tank1/3(E1)
  CT3/1 -> Tank3/1(CT3)
  EB3/1 -> Tank3/3(EB3)
  T3/1 -> Tank3/2(T3)
  CT1/1 -> Tank1/1(CT1)

== system c00014M_harness/M237 ==
  note: VALUES
      | ---------------------------------
      | ControlType = 1 | 2 | 3
      | FillTank = 0 | 1
      | EmptyTank = 0 | 1
      | ManualReference between 0 and 1
      | Tempreature between 0 and 100
      | EmergencyButton = 0 | 1
      | LiquidLevel between 0 and 1 (hmax)
  note: Inputs For Tank2
  note: NAMES
      | --------------------------------------------
      | CT1 = ControlType Tank 1
      | F1 = Fill Tank 1
      | E1 = Empty Tank 1
      | MR1 = Manual Reference Tank1
      | T1 = Temperature Tank 1
      | EB1 = Emergency Button Tank 1
      | LL1 = Liquid Level 1
  note: Inputs For Tank3
  note: Inputs For Tank1
  CT1 : Inport
  F1 : Inport  Port=2
  E1 : Inport  Port=3
  T1 : Inport  Port=4
  EB1 : Inport  Port=5
  CT3 : Inport  Port=6
  T3 : Inport  Port=7
  EB3 : Inport  Port=8
  Tank1 : Subsystem
  Tank3 : Subsystem
  LL1 : Outport
  LL3 : Outport  Port=2
  wires:
  EB1/1 -> Tank1/5(EB1)
  Tank3/1(LL3) -> LL3/1, Tank1/6(LL3)
  T1/1 -> Tank1/4(T1)
  Tank1/1(LL1) -> LL1/1, Tank3/4(LL1)
  F1/1 -> Tank1/2(F1)
  E1/1 -> Tank1/3(E1)
  CT3/1 -> Tank3/1(CT3)
  EB3/1 -> Tank3/3(EB3)
  T3/1 -> Tank3/2(T3)
  CT1/1 -> Tank1/1(CT1)

== system c00014M_harness/M238 ==
  note: VALUES
      | ---------------------------------
      | ControlType = 1 | 2 | 3
      | FillTank = 0 | 1
      | EmptyTank = 0 | 1
      | ManualReference between 0 and 1
      | Tempreature between 0 and 100
      | EmergencyButton = 0 | 1
      | LiquidLevel between 0 and 1 (hmax)
  note: Inputs For Tank2
  note: NAMES
      | --------------------------------------------
      | CT1 = ControlType Tank 1
      | F1 = Fill Tank 1
      | E1 = Empty Tank 1
      | MR1 = Manual Reference Tank1
      | T1 = Temperature Tank 1
      | EB1 = Emergency Button Tank 1
      | LL1 = Liquid Level 1
  note: Inputs For Tank3
  note: Inputs For Tank1
  CT1 : Inport
  F1 : Inport  Port=2
  E1 : Inport  Port=3
  T1 : Inport  Port=4
  EB1 : Inport  Port=5
  CT3 : Inport  Port=6
  T3 : Inport  Port=7
  EB3 : Inport  Port=8
  Tank1 : Subsystem
  Tank3 : Subsystem
  LL1 : Outport
  LL3 : Outport  Port=2
  wires:
  EB1/1 -> Tank1/5(EB1)
  Tank3/1(LL3) -> LL3/1, Tank1/6(LL3)
  T1/1 -> Tank1/4(T1)
  Tank1/1(LL1) -> LL1/1, Tank3/4(LL1)
  F1/1 -> Tank1/2(F1)
  E1/1 -> Tank1/3(E1)
  CT3/1 -> Tank3/1(CT3)
  EB3/1 -> Tank3/3(EB3)
  T3/1 -> Tank3/2(T3)
  CT1/1 -> Tank1/1(CT1)

== system c00014M_harness/M239 ==
  note: VALUES
      | ---------------------------------
      | ControlType = 1 | 2 | 3
      | FillTank = 0 | 1
      | EmptyTank = 0 | 1
      | ManualReference between 0 and 1
      | Tempreature between 0 and 100
      | EmergencyButton = 0 | 1
      | LiquidLevel between 0 and 1 (hmax)
  note: Inputs For Tank2
  note: NAMES
      | --------------------------------------------
      | CT1 = ControlType Tank 1
      | F1 = Fill Tank 1
      | E1 = Empty Tank 1
      | MR1 = Manual Reference Tank1
      | T1 = Temperature Tank 1
      | EB1 = Emergency Button Tank 1
      | LL1 = Liquid Level 1
  note: Inputs For Tank3
  note: Inputs For Tank1
  CT1 : Inport
  F1 : Inport  Port=2
  E1 : Inport  Port=3
  T1 : Inport  Port=4
  EB1 : Inport  Port=5
  CT3 : Inport  Port=6
  T3 : Inport  Port=7
  EB3 : Inport  Port=8
  Tank1 : Subsystem
  Tank3 : Subsystem
  LL1 : Outport
  LL3 : Outport  Port=2
  wires:
  EB1/1 -> Tank1/5(EB1)
  Tank3/1(LL3) -> LL3/1, Tank1/6(LL3)
  T1/1 -> Tank1/4(T1)
  Tank1/1(LL1) -> LL1/1, Tank3/4(LL1)
  F1/1 -> Tank1/2(F1)
  E1/1 -> Tank1/3(E1)
  CT3/1 -> Tank3/1(CT3)
  EB3/1 -> Tank3/3(EB3)
  T3/1 -> Tank3/2(T3)
  CT1/1 -> Tank1/1(CT1)

== system c00014M_harness/M240 ==
  note: VALUES
      | ---------------------------------
      | ControlType = 1 | 2 | 3
      | FillTank = 0 | 1
      | EmptyTank = 0 | 1
      | ManualReference between 0 and 1
      | Tempreature between 0 and 100
      | EmergencyButton = 0 | 1
      | LiquidLevel between 0 and 1 (hmax)
  note: Inputs For Tank2
  note: NAMES
      | --------------------------------------------
      | CT1 = ControlType Tank 1
      | F1 = Fill Tank 1
      | E1 = Empty Tank 1
      | MR1 = Manual Reference Tank1
      | T1 = Temperature Tank 1
      | EB1 = Emergency Button Tank 1
      | LL1 = Liquid Level 1
  note: Inputs For Tank3
  note: Inputs For Tank1
  CT1 : Inport
  F1 : Inport  Port=2
  E1 : Inport  Port=3
  T1 : Inport  Port=4
  EB1 : Inport  Port=5
  CT3 : Inport  Port=6
  T3 : Inport  Port=7
  EB3 : Inport  Port=8
  Tank1 : Subsystem
  Tank3 : Subsystem
  LL1 : Outport
  LL3 : Outport  Port=2
  wires:
  EB1/1 -> Tank1/5(EB1)
  Tank3/1(LL3) -> LL3/1, Tank1/6(LL3)
  T1/1 -> Tank1/4(T1)
  Tank1/1(LL1) -> LL1/1, Tank3/4(LL1)
  F1/1 -> Tank1/2(F1)
  E1/1 -> Tank1/3(E1)
  CT3/1 -> Tank3/1(CT3)
  EB3/1 -> Tank3/3(EB3)
  T3/1 -> Tank3/2(T3)
  CT1/1 -> Tank1/1(CT1)

== system c00014M_harness/M241 ==
  note: VALUES
      | ---------------------------------
      | ControlType = 1 | 2 | 3
      | FillTank = 0 | 1
      | EmptyTank = 0 | 1
      | ManualReference between 0 and 1
      | Tempreature between 0 and 100
      | EmergencyButton = 0 | 1
      | LiquidLevel between 0 and 1 (hmax)
  note: Inputs For Tank2
  note: NAMES
      | --------------------------------------------
      | CT1 = ControlType Tank 1
      | F1 = Fill Tank 1
      | E1 = Empty Tank 1
      | MR1 = Manual Reference Tank1
      | T1 = Temperature Tank 1
      | EB1 = Emergency Button Tank 1
      | LL1 = Liquid Level 1
  note: Inputs For Tank3
  note: Inputs For Tank1
  CT1 : Inport
  F1 : Inport  Port=2
  E1 : Inport  Port=3
  T1 : Inport  Port=4
  EB1 : Inport  Port=5
  CT3 : Inport  Port=6
  T3 : Inport  Port=7
  EB3 : Inport  Port=8
  Tank1 : Subsystem
  Tank3 : Subsystem
  LL1 : Outport
  LL3 : Outport  Port=2
  wires:
  EB1/1 -> Tank1/5(EB1)
  Tank3/1(LL3) -> LL3/1, Tank1/6(LL3)
  T1/1 -> Tank1/4(T1)
  Tank1/1(LL1) -> LL1/1, Tank3/4(LL1)
  F1/1 -> Tank1/2(F1)
  E1/1 -> Tank1/3(E1)
  CT3/1 -> Tank3/1(CT3)
  EB3/1 -> Tank3/3(EB3)
  T3/1 -> Tank3/2(T3)
  CT1/1 -> Tank1/1(CT1)

== system c00014M_harness/M242 ==
  note: VALUES
      | ---------------------------------
      | ControlType = 1 | 2 | 3
      | FillTank = 0 | 1
      | EmptyTank = 0 | 1
      | ManualReference between 0 and 1
      | Tempreature between 0 and 100
      | EmergencyButton = 0 | 1
      | LiquidLevel between 0 and 1 (hmax)
  note: Inputs For Tank2
  note: NAMES
      | --------------------------------------------
      | CT1 = ControlType Tank 1
      | F1 = Fill Tank 1
      | E1 = Empty Tank 1
      | MR1 = Manual Reference Tank1
      | T1 = Temperature Tank 1
      | EB1 = Emergency Button Tank 1
      | LL1 = Liquid Level 1
  note: Inputs For Tank3
  note: Inputs For Tank1
  CT1 : Inport
  F1 : Inport  Port=2
  E1 : Inport  Port=3
  T1 : Inport  Port=4
  EB1 : Inport  Port=5
  CT3 : Inport  Port=6
  T3 : Inport  Port=7
  EB3 : Inport  Port=8
  Tank1 : Subsystem
  Tank3 : Subsystem
  LL1 : Outport
  LL3 : Outport  Port=2
  wires:
  EB1/1 -> Tank1/5(EB1)
  Tank3/1(LL3) -> LL3/1, Tank1/6(LL3)
  T1/1 -> Tank1/4(T1)
  Tank1/1(LL1) -> LL1/1, Tank3/4(LL1)
  F1/1 -> Tank1/2(F1)
  E1/1 -> Tank1/3(E1)
  CT3/1 -> Tank3/1(CT3)
  EB3/1 -> Tank3/3(EB3)
  T3/1 -> Tank3/2(T3)
  CT1/1 -> Tank1/1(CT1)

== system c00014M_harness/M243 ==
  note: VALUES
      | ---------------------------------
      | ControlType = 1 | 2 | 3
      | FillTank = 0 | 1
      | EmptyTank = 0 | 1
      | ManualReference between 0 and 1
      | Tempreature between 0 and 100
      | EmergencyButton = 0 | 1
      | LiquidLevel between 0 and 1 (hmax)
  note: Inputs For Tank2
  note: NAMES
      | --------------------------------------------
      | CT1 = ControlType Tank 1
      | F1 = Fill Tank 1
      | E1 = Empty Tank 1
      | MR1 = Manual Reference Tank1
      | T1 = Temperature Tank 1
      | EB1 = Emergency Button Tank 1
      | LL1 = Liquid Level 1
  note: Inputs For Tank3
  note: Inputs For Tank1
  CT1 : Inport
  F1 : Inport  Port=2
  E1 : Inport  Port=3
  T1 : Inport  Port=4
  EB1 : Inport  Port=5
  CT3 : Inport  Port=6
  T3 : Inport  Port=7
  EB3 : Inport  Port=8
  Tank1 : Subsystem
  Tank3 : Subsystem
  LL1 : Outport
  LL3 : Outport  Port=2
  wires:
  EB1/1 -> Tank1/5(EB1)
  Tank3/1(LL3) -> LL3/1, Tank1/6(LL3)
  T1/1 -> Tank1/4(T1)
  Tank1/1(LL1) -> LL1/1, Tank3/4(LL1)
  F1/1 -> Tank1/2(F1)
  E1/1 -> Tank1/3(E1)
  CT3/1 -> Tank3/1(CT3)
  EB3/1 -> Tank3/3(EB3)
  T3/1 -> Tank3/2(T3)
  CT1/1 -> Tank1/1(CT1)

== system c00014M_harness/M244 ==
  note: VALUES
      | ---------------------------------
      | ControlType = 1 | 2 | 3
      | FillTank = 0 | 1
      | EmptyTank = 0 | 1
      | ManualReference between 0 and 1
      | Tempreature between 0 and 100
      | EmergencyButton = 0 | 1
      | LiquidLevel between 0 and 1 (hmax)
  note: Inputs For Tank2
  note: NAMES
      | --------------------------------------------
      | CT1 = ControlType Tank 1
      | F1 = Fill Tank 1
      | E1 = Empty Tank 1
      | MR1 = Manual Reference Tank1
      | T1 = Temperature Tank 1
      | EB1 = Emergency Button Tank 1
      | LL1 = Liquid Level 1
  note: Inputs For Tank3
  note: Inputs For Tank1
  CT1 : Inport
  F1 : Inport  Port=2
  E1 : Inport  Port=3
  T1 : Inport  Port=4
  EB1 : Inport  Port=5
  CT3 : Inport  Port=6
  T3 : Inport  Port=7
  EB3 : Inport  Port=8
  Tank1 : Subsystem
  Tank3 : Subsystem
  LL1 : Outport
  LL3 : Outport  Port=2
  wires:
  EB1/1 -> Tank1/5(EB1)
  Tank3/1(LL3) -> LL3/1, Tank1/6(LL3)
  T1/1 -> Tank1/4(T1)
  Tank1/1(LL1) -> LL1/1, Tank3/4(LL1)
  F1/1 -> Tank1/2(F1)
  E1/1 -> Tank1/3(E1)
  CT3/1 -> Tank3/1(CT3)
  EB3/1 -> Tank3/3(EB3)
  T3/1 -> Tank3/2(T3)
  CT1/1 -> Tank1/1(CT1)

== system c00014M_harness/M245 ==
  note: VALUES
      | ---------------------------------
      | ControlType = 1 | 2 | 3
      | FillTank = 0 | 1
      | EmptyTank = 0 | 1
      | ManualReference between 0 and 1
      | Tempreature between 0 and 100
      | EmergencyButton = 0 | 1
      | LiquidLevel between 0 and 1 (hmax)
  note: Inputs For Tank2
  note: NAMES
      | --------------------------------------------
      | CT1 = ControlType Tank 1
      | F1 = Fill Tank 1
      | E1 = Empty Tank 1
      | MR1 = Manual Reference Tank1
      | T1 = Temperature Tank 1
      | EB1 = Emergency Button Tank 1
      | LL1 = Liquid Level 1
  note: Inputs For Tank3
  note: Inputs For Tank1
  CT1 : Inport
  F1 : Inport  Port=2
  E1 : Inport  Port=3
  T1 : Inport  Port=4
  EB1 : Inport  Port=5
  CT3 : Inport  Port=6
  T3 : Inport  Port=7
  EB3 : Inport  Port=8
  Tank1 : Subsystem
  Tank3 : Subsystem
  LL1 : Outport
  LL3 : Outport  Port=2
  wires:
  EB1/1 -> Tank1/5(EB1)
  Tank3/1(LL3) -> LL3/1, Tank1/6(LL3)
  T1/1 -> Tank1/4(T1)
  Tank1/1(LL1) -> LL1/1, Tank3/4(LL1)
  F1/1 -> Tank1/2(F1)
  E1/1 -> Tank1/3(E1)
  CT3/1 -> Tank3/1(CT3)
  EB3/1 -> Tank3/3(EB3)
  T3/1 -> Tank3/2(T3)
  CT1/1 -> Tank1/1(CT1)

== system c00014M_harness/M246 ==
  note: VALUES
      | ---------------------------------
      | ControlType = 1 | 2 | 3
      | FillTank = 0 | 1
      | EmptyTank = 0 | 1
      | ManualReference between 0 and 1
      | Tempreature between 0 and 100
      | EmergencyButton = 0 | 1
      | LiquidLevel between 0 and 1 (hmax)
  note: Inputs For Tank2
  note: NAMES
      | --------------------------------------------
      | CT1 = ControlType Tank 1
      | F1 = Fill Tank 1
      | E1 = Empty Tank 1
      | MR1 = Manual Reference Tank1
      | T1 = Temperature Tank 1
      | EB1 = Emergency Button Tank 1
      | LL1 = Liquid Level 1
  note: Inputs For Tank3
  note: Inputs For Tank1
  CT1 : Inport
  F1 : Inport  Port=2
  E1 : Inport  Port=3
  T1 : Inport  Port=4
  EB1 : Inport  Port=5
  CT3 : Inport  Port=6
  T3 : Inport  Port=7
  EB3 : Inport  Port=8
  Tank1 : Subsystem
  Tank3 : Subsystem
  LL1 : Outport
  LL3 : Outport  Port=2
  wires:
  EB1/1 -> Tank1/5(EB1)
  Tank3/1(LL3) -> LL3/1, Tank1/6(LL3)
  T1/1 -> Tank1/4(T1)
  Tank1/1(LL1) -> LL1/1, Tank3/4(LL1)
  F1/1 -> Tank1/2(F1)
  E1/1 -> Tank1/3(E1)
  CT3/1 -> Tank3/1(CT3)
  EB3/1 -> Tank3/3(EB3)
  T3/1 -> Tank3/2(T3)
  CT1/1 -> Tank1/1(CT1)

== system c00014M_harness/CPSUT/Tank1 ==
  CT1 : Inport
  F1 : Inport  Port=2
  E1 : Inport  Port=3
  T1 : Inport  Port=4
  EB1 : Inport  Port=5
  LL3 : Inport  Port=6
  Control : Subsystem
  Logical Operator : Logic  AllPortsSameDT=off  OutDataTypeStr=boolean
  MasterTankControl : Subsystem
  Memory : Memory
  Memory2 : Memory
  TankModel : Subsystem
  LL1 : Outport
  wires:
  TankModel/1(LiquidLevel) -> Memory/1, LL1/1
  Control/1(LiquidIn) -> Logical Operator/1
  Control/2(LiquidOut) -> TankModel/2(LiquidOut)
  Memory/1 -> Control/5(LiquidLevel), MasterTankControl/1(LiquidTank1)
  CT1/1 -> Control/1(ControlType)
  F1/1 -> Control/2(Fill)
  E1/1 -> Control/3(Empty)
  LL3/1 -> Memory2/1
  Memory2/1 -> MasterTankControl/2(LiquidTank3)
  EB1/1 -> Control/4(EmergencyButton)
  MasterTankControl/1(AllowTheTankFilling) -> Logical Operator/2
  Logical Operator/1 -> TankModel/1(LiquidIn)

== system c00014M_harness/CPSUT/Tank3 ==
  CT3 : Inport
  T3 : Inport  Port=2
  EB3 : Inport  Port=3
  LL1 : Inport  Port=4
  Control : Subsystem
  Logical Operator : Logic  AllPortsSameDT=off  OutDataTypeStr=boolean
  MasterTankControl : Subsystem
  Memory : Memory
  Memory1 : Memory
  TankModel : Subsystem
  LL3 : Outport
  wires:
  TankModel/1(LiquidLevel) -> Memory/1, LL3/1
  Control/1(LiquidIn) -> Logical Operator/1
  Control/2(LiquidOut) -> TankModel/2(LiquidOut)
  Memory/1 -> MasterTankControl/2(LiquidTank3), Control/4(LiquidLevel)
  CT3/1 -> Control/2(StartMaintenance), Control/1(ControlType)
  Memory1/1 -> MasterTankControl/1(LiquidTank1)
  EB3/1 -> Control/3(EmergencyButton)
  MasterTankControl/1(AllowTheTankFilling) -> Logical Operator/2
  Logical Operator/1 -> TankModel/1(LiquidIn)
  LL1/1 -> Memory1/1

== system c00014M_harness/M001/Tank1 ==
  CT1 : Inport
  F1 : Inport  Port=2
  E1 : Inport  Port=3
  T1 : Inport  Port=4
  EB1 : Inport  Port=5
  LL3 : Inport  Port=6
  Control : Subsystem
  Logical Operator : Logic  AllPortsSameDT=off  OutDataTypeStr=boolean
  MasterTankControl : Subsystem
  Memory : Memory
  Memory2 : Memory
  TankModel : Subsystem
  LL1 : Outport
  wires:
  Logical Operator/1 -> TankModel/1(LiquidIn)
  MasterTankControl/1(AllowTheTankFilling) -> Logical Operator/2
  EB1/1 -> Control/4(EmergencyButton)
  Memory2/1 -> MasterTankControl/2(LiquidTank3)
  LL3/1 -> Memory2/1
  E1/1 -> Control/3(Empty)
  F1/1 -> Control/2(Fill)
  CT1/1 -> Control/1(ControlType)
  Memory/1 -> MasterTankControl/1(LiquidTank1), Control/5(LiquidLevel)
  Control/2(LiquidOut) -> TankModel/2(LiquidOut)
  Control/1(LiquidIn) -> Logical Operator/1
  TankModel/1(LiquidLevel) -> LL1/1, Memory/1

== system c00014M_harness/M001/Tank3 ==
  CT3 : Inport
  T3 : Inport  Port=2
  EB3 : Inport  Port=3
  LL1 : Inport  Port=4
  Control : Subsystem
  Logical Operator : Logic  AllPortsSameDT=off  OutDataTypeStr=boolean
  MasterTankControl : Subsystem
  Memory : Memory
  Memory1 : Memory
  TankModel : Subsystem
  LL3 : Outport
  wires:
  LL1/1 -> Memory1/1
  Logical Operator/1 -> TankModel/1(LiquidIn)
  MasterTankControl/1(AllowTheTankFilling) -> Logical Operator/2
  EB3/1 -> Control/3(EmergencyButton)
  Memory1/1 -> MasterTankControl/1(LiquidTank1)
  CT3/1 -> Control/1(ControlType), Control/2(StartMaintenance)
  Memory/1 -> Control/4(LiquidLevel), MasterTankControl/2(LiquidTank3)
  Control/2(LiquidOut) -> TankModel/2(LiquidOut)
  Control/1(LiquidIn) -> Logical Operator/1
  TankModel/1(LiquidLevel) -> LL3/1, Memory/1

== system c00014M_harness/M036/Tank1 ==
  CT1 : Inport
  F1 : Inport  Port=2
  E1 : Inport  Port=3
  T1 : Inport  Port=4
  EB1 : Inport  Port=5
  LL3 : Inport  Port=6
  Control : Subsystem
  Logical Operator : Logic  AllPortsSameDT=off  OutDataTypeStr=boolean
  MasterTankControl : Subsystem
  Memory : Memory
  Memory2 : Memory
  TankModel : Subsystem
  LL1 : Outport
  wires:
  TankModel/1(LiquidLevel) -> Memory/1, LL1/1
  Control/1(LiquidIn) -> Logical Operator/1
  Control/2(LiquidOut) -> TankModel/2(LiquidOut)
  Memory/1 -> Control/5(LiquidLevel), MasterTankControl/1(LiquidTank1)
  CT1/1 -> Control/1(ControlType)
  F1/1 -> Control/2(Fill)
  E1/1 -> Control/3(Empty)
  LL3/1 -> Memory2/1
  Memory2/1 -> MasterTankControl/2(LiquidTank3)
  EB1/1 -> Control/4(EmergencyButton)
  MasterTankControl/1(AllowTheTankFilling) -> Logical Operator/2
  Logical Operator/1 -> TankModel/1(LiquidIn)

== system c00014M_harness/M036/Tank3 ==
  CT3 : Inport
  T3 : Inport  Port=2
  EB3 : Inport  Port=3
  LL1 : Inport  Port=4
  Control : Subsystem
  Logical Operator : Logic  AllPortsSameDT=off  OutDataTypeStr=boolean
  MasterTankControl : Subsystem
  Memory : Memory
  Memory1 : Memory
  TankModel : Subsystem
  LL3 : Outport
  wires:
  TankModel/1(LiquidLevel) -> Memory/1, LL3/1
  Control/1(LiquidIn) -> Logical Operator/1
  Control/2(LiquidOut) -> TankModel/2(LiquidOut)
  Memory/1 -> MasterTankControl/2(LiquidTank3), Control/4(LiquidLevel)
  CT3/1 -> Control/2(StartMaintenance), Control/1(ControlType)
  Memory1/1 -> MasterTankControl/1(LiquidTank1)
  EB3/1 -> Control/3(EmergencyButton)
  MasterTankControl/1(AllowTheTankFilling) -> Logical Operator/2
  Logical Operator/1 -> TankModel/1(LiquidIn)
  LL1/1 -> Memory1/1
